simulink library "mylib"  (R2020a)
settings: Solver=VariableStepAuto  StartTime=0.0  StopTime=10.0  RelTol=1e-3
undefined symbols (not defined in the file): d_du_max_pu, dir_to_bus1, dir_to_bus_0L, dir_to_bus_2, dir_to_line1, dir_to_line_0L, dir_to_line_2, du_max_pu, du_ph_max_pu, Fi_0, Fi_T_H, Fi_T_L, Fi_T_M, I0_calc_0L, I0_comp_H, I0_comp_L, I0_comp_M, I0_max_0L, I2_max_2, I_diff1, I_diff2, I_diff3, I_diff4, I_diff5, I_diff_to, I_hight_CT1_G, I_hight_CT2_G, I_low_CT1, I_low_CT2, I_max1, I_max2, I_max3, I_max4, I_max5, I_min_sec_CT1, I_min_sec_CT2, I_unb, Iph_max_0L, Iph_max_2, jmp_in_zone, jmp_in_zone_0L, jmp_in_zone_2, K_dop, max_min1, only_K1_0L, only_K1_2, only_K2_0L, only_K2_2, only_K3_0L, only_K3_2, P_ctl_0, PQ_Fi_ctl_0, Q_ctl_0, S_set_0, set, set1, T_fast, T_I_ctl, T_off, T_on ... (+15)
libraries: $bdroot x184, powerlib_meascontrol x97
(part 11 of 14)

== system mylib/264_DZ_trans_st_v1/Poly12_det19_ph/Zc/stp_12 ==
  Y_in : Inport
  alg_in : Inport  Port=2
  Re_cur : Inport  Port=3
  Im_cur : Inport  Port=4
  Re_next : Inport  Port=5
  Im_next : Inport  Port=6
  re : Inport  Port=7
  im : Inport  Port=8
  start_pt : Inport  Port=9
  Re_start : Inport  Port=10
  Im_start : Inport  Port=11
  Constant : Constant  Value=0
  Constant1 : Constant  Value=0
  D1 : Logic  AllPortsSameDT=off  OutDataTypeStr=boolean
  Divide : Product  Inputs=**
  Divide1 : Product  Inputs=*/
  Logical Operator1 : Logic  Inputs=3  AllPortsSameDT=off  OutDataTypeStr=boolean
  Logical Operator2 : Logic  AllPortsSameDT=off  OutDataTypeStr=boolean
  Logical Operator3 : Logic  AllPortsSameDT=off  OutDataTypeStr=boolean
  Logical Operator4 : Logic  Operator=OR  AllPortsSameDT=off  OutDataTypeStr=boolean
  Logical Operator5 : Logic  AllPortsSameDT=off  OutDataTypeStr=boolean
  Logical Operator6 : Logic  Operator=OR  AllPortsSameDT=off  OutDataTypeStr=boolean
  Logical Operator7 : Logic  Operator=NOT  AllPortsSameDT=off  OutDataTypeStr=boolean
  Logical Operator8 : Logic  Operator=NOT  AllPortsSameDT=off  OutDataTypeStr=boolean
  Relational Operator{,1..3} (4 alike) : RelationalOperator  Operator===  OutDataTypeStr=boolean  RndMeth=Simplest
  Relational Operator4 : RelationalOperator  Operator=<  OutDataTypeStr=boolean  RndMeth=Simplest
  Relational Operator5 : RelationalOperator  Operator=>  OutDataTypeStr=boolean  RndMeth=Simplest
  Relational Operator6 : RelationalOperator  Operator=<  OutDataTypeStr=boolean  RndMeth=Simplest
  Relational Operator7 : RelationalOperator  Operator=>  OutDataTypeStr=boolean  RndMeth=Simplest
  Relational Operator8 : RelationalOperator  Operator=>  OutDataTypeStr=boolean  RndMeth=Simplest
  Switch{1..6} (6 alike) : Switch  Criteria=u2 > Threshold
  X2-X1 : Sum  Inputs=+-
  Y-Y1 : Sum  Inputs=+-
  Y2-Y1 : Sum  Inputs=+-
  Y2-Y2 : Sum
  Y_out : Outport
  alg_out : Outport  Port=2
  cur_Re : Outport  Port=3
  cur_Im : Outport  Port=4
  wires:
  Constant/1 -> Relational Operator1/2, Relational Operator/2
  Relational Operator1/1 -> D1/1
  Relational Operator/1 -> D1/2
  D1/1 -> Logical Operator1/1, Switch1/2, Switch2/2
  Re_next/1 -> Switch2/3, Relational Operator1/1
  Im_next/1 -> Switch1/3, Relational Operator/1
  Constant1/1 -> Relational Operator3/2, Relational Operator2/2
  Relational Operator2/1 -> Logical Operator1/3
  Relational Operator3/1 -> Logical Operator1/2
  Relational Operator4/1 -> Logical Operator2/1
  Relational Operator5/1 -> Logical Operator2/2
  Relational Operator6/1 -> Logical Operator3/1
  Relational Operator7/1 -> Logical Operator3/2
  Logical Operator2/1 -> Logical Operator4/1
  Logical Operator3/1 -> Logical Operator4/2
  Logical Operator4/1 -> Logical Operator5/1
  Logical Operator1/1 -> Logical Operator7/1
  Logical Operator7/1 -> Logical Operator6/1
  start_pt/1 -> Logical Operator6/2
  X2-X1/1 -> Divide/2
  Divide/1 -> Divide1/1
  Y2-Y1/1 -> Divide1/2
  Y-Y1/1 -> Divide/1
  Divide1/1 -> Y2-Y2/1
  Re_cur/1 -> Relational Operator3/1, X2-X1/2, Switch5/3, Y2-Y2/2
  Im_start/1 -> Switch1/1
  Re_start/1 -> Switch2/1
  re/1 -> Relational Operator8/2
  Y2-Y2/1 -> Relational Operator8/1
  im/1 -> Relational Operator7/1, Relational Operator6/1, Relational Operator5/1, Relational Operator4/1, Y-Y1/1
  Im_cur/1 -> Y2-Y1/2, Y-Y1/2, Relational Operator2/1, Switch6/3, Relational Operator6/2, Relational Operator5/2
  Switch2/1 -> X2-X1/1, Switch5/1
  Switch1/1 -> Y2-Y1/1, Switch6/1, Relational Operator7/2, Relational Operator4/2
  Relational Operator8/1 -> Logical Operator5/2
  Logical Operator5/1 -> Switch3/2
  Logical Operator6/1 -> Switch6/2, Switch5/2, Switch4/2
  Y_in/1 -> Switch4/3
  Switch3/1 -> alg_out/1, Switch4/1
  alg_in/1 -> Logical Operator8/1, Switch3/3
  Logical Operator8/1 -> Switch3/1
  Switch4/1 -> Y_out/1
  Switch6/1 -> cur_Im/1
  Switch5/1 -> cur_Re/1

== system mylib/264_DZ_trans_st_v1/Poly12_det19_ph/Zc/stp_2 ==
  Y_in : Inport
  alg_in : Inport  Port=2
  Re_cur : Inport  Port=3
  Im_cur : Inport  Port=4
  Re_next : Inport  Port=5
  Im_next : Inport  Port=6
  re : Inport  Port=7
  im : Inport  Port=8
  start_pt : Inport  Port=9
  Re_start : Inport  Port=10
  Im_start : Inport  Port=11
  Constant : Constant  Value=0
  Constant1 : Constant  Value=0
  D1 : Logic  AllPortsSameDT=off  OutDataTypeStr=boolean
  Divide : Product  Inputs=**
  Divide1 : Product  Inputs=*/
  Logical Operator1 : Logic  Inputs=3  AllPortsSameDT=off  OutDataTypeStr=boolean
  Logical Operator2 : Logic  AllPortsSameDT=off  OutDataTypeStr=boolean
  Logical Operator3 : Logic  AllPortsSameDT=off  OutDataTypeStr=boolean
  Logical Operator4 : Logic  Operator=OR  AllPortsSameDT=off  OutDataTypeStr=boolean
  Logical Operator5 : Logic  AllPortsSameDT=off  OutDataTypeStr=boolean
  Logical Operator6 : Logic  Operator=OR  AllPortsSameDT=off  OutDataTypeStr=boolean
  Logical Operator7 : Logic  Operator=NOT  AllPortsSameDT=off  OutDataTypeStr=boolean
  Logical Operator8 : Logic  Operator=NOT  AllPortsSameDT=off  OutDataTypeStr=boolean
  Relational Operator{,1..3} (4 alike) : RelationalOperator  Operator===  OutDataTypeStr=boolean  RndMeth=Simplest
  Relational Operator4 : RelationalOperator  Operator=<  OutDataTypeStr=boolean  RndMeth=Simplest
  Relational Operator5 : RelationalOperator  Operator=>  OutDataTypeStr=boolean  RndMeth=Simplest
  Relational Operator6 : RelationalOperator  Operator=<  OutDataTypeStr=boolean  RndMeth=Simplest
  Relational Operator7 : RelationalOperator  Operator=>  OutDataTypeStr=boolean  RndMeth=Simplest
  Relational Operator8 : RelationalOperator  Operator=>  OutDataTypeStr=boolean  RndMeth=Simplest
  Switch{1..6} (6 alike) : Switch  Criteria=u2 > Threshold
  X2-X1 : Sum  Inputs=+-
  Y-Y1 : Sum  Inputs=+-
  Y2-Y1 : Sum  Inputs=+-
  Y2-Y2 : Sum
  Y_out : Outport
  alg_out : Outport  Port=2
  cur_Re : Outport  Port=3
  cur_Im : Outport  Port=4
  wires:
  Constant/1 -> Relational Operator1/2, Relational Operator/2
  Relational Operator1/1 -> D1/1
  Relational Operator/1 -> D1/2
  D1/1 -> Logical Operator1/1, Switch1/2, Switch2/2
  Re_next/1 -> Switch2/3, Relational Operator1/1
  Im_next/1 -> Switch1/3, Relational Operator/1
  Constant1/1 -> Relational Operator3/2, Relational Operator2/2
  Relational Operator2/1 -> Logical Operator1/3
  Relational Operator3/1 -> Logical Operator1/2
  Relational Operator4/1 -> Logical Operator2/1
  Relational Operator5/1 -> Logical Operator2/2
  Relational Operator6/1 -> Logical Operator3/1
  Relational Operator7/1 -> Logical Operator3/2
  Logical Operator2/1 -> Logical Operator4/1
  Logical Operator3/1 -> Logical Operator4/2
  Logical Operator4/1 -> Logical Operator5/1
  Logical Operator1/1 -> Logical Operator7/1
  Logical Operator7/1 -> Logical Operator6/1
  start_pt/1 -> Logical Operator6/2
  X2-X1/1 -> Divide/2
  Divide/1 -> Divide1/1
  Y2-Y1/1 -> Divide1/2
  Y-Y1/1 -> Divide/1
  Divide1/1 -> Y2-Y2/1
  Re_cur/1 -> Relational Operator3/1, X2-X1/2, Switch5/3, Y2-Y2/2
  Im_start/1 -> Switch1/1
  Re_start/1 -> Switch2/1
  re/1 -> Relational Operator8/2
  Y2-Y2/1 -> Relational Operator8/1
  im/1 -> Relational Operator7/1, Relational Operator6/1, Relational Operator5/1, Relational Operator4/1, Y-Y1/1
  Im_cur/1 -> Y2-Y1/2, Y-Y1/2, Relational Operator2/1, Switch6/3, Relational Operator6/2, Relational Operator5/2
  Switch2/1 -> X2-X1/1, Switch5/1
  Switch1/1 -> Y2-Y1/1, Switch6/1, Relational Operator7/2, Relational Operator4/2
  Relational Operator8/1 -> Logical Operator5/2
  Logical Operator5/1 -> Switch3/2
  Logical Operator6/1 -> Switch6/2, Switch5/2, Switch4/2
  Y_in/1 -> Switch4/3
  Switch3/1 -> alg_out/1, Switch4/1
  alg_in/1 -> Logical Operator8/1, Switch3/3
  Logical Operator8/1 -> Switch3/1
  Switch4/1 -> Y_out/1
  Switch6/1 -> cur_Im/1
  Switch5/1 -> cur_Re/1

== system mylib/264_DZ_trans_st_v1/Poly12_det19_ph/Zc/stp_3 ==
  Y_in : Inport
  alg_in : Inport  Port=2
  Re_cur : Inport  Port=3
  Im_cur : Inport  Port=4
  Re_next : Inport  Port=5
  Im_next : Inport  Port=6
  re : Inport  Port=7
  im : Inport  Port=8
  start_pt : Inport  Port=9
  Re_start : Inport  Port=10
  Im_start : Inport  Port=11
  Constant : Constant  Value=0
  Constant1 : Constant  Value=0
  D1 : Logic  AllPortsSameDT=off  OutDataTypeStr=boolean
  Divide : Product  Inputs=**
  Divide1 : Product  Inputs=*/
  Logical Operator1 : Logic  Inputs=3  AllPortsSameDT=off  OutDataTypeStr=boolean
  Logical Operator2 : Logic  AllPortsSameDT=off  OutDataTypeStr=boolean
  Logical Operator3 : Logic  AllPortsSameDT=off  OutDataTypeStr=boolean
  Logical Operator4 : Logic  Operator=OR  AllPortsSameDT=off  OutDataTypeStr=boolean
  Logical Operator5 : Logic  AllPortsSameDT=off  OutDataTypeStr=boolean
  Logical Operator6 : Logic  Operator=OR  AllPortsSameDT=off  OutDataTypeStr=boolean
  Logical Operator7 : Logic  Operator=NOT  AllPortsSameDT=off  OutDataTypeStr=boolean
  Logical Operator8 : Logic  Operator=NOT  AllPortsSameDT=off  OutDataTypeStr=boolean
  Relational Operator{,1..3} (4 alike) : RelationalOperator  Operator===  OutDataTypeStr=boolean  RndMeth=Simplest
  Relational Operator4 : RelationalOperator  Operator=<  OutDataTypeStr=boolean  RndMeth=Simplest
  Relational Operator5 : RelationalOperator  Operator=>  OutDataTypeStr=boolean  RndMeth=Simplest
  Relational Operator6 : RelationalOperator  Operator=<  OutDataTypeStr=boolean  RndMeth=Simplest
  Relational Operator7 : RelationalOperator  Operator=>  OutDataTypeStr=boolean  RndMeth=Simplest
  Relational Operator8 : RelationalOperator  Operator=>  OutDataTypeStr=boolean  RndMeth=Simplest
  Switch{1..6} (6 alike) : Switch  Criteria=u2 > Threshold
  X2-X1 : Sum  Inputs=+-
  Y-Y1 : Sum  Inputs=+-
  Y2-Y1 : Sum  Inputs=+-
  Y2-Y2 : Sum
  Y_out : Outport
  alg_out : Outport  Port=2
  cur_Re : Outport  Port=3
  cur_Im : Outport  Port=4
  wires:
  Constant/1 -> Relational Operator1/2, Relational Operator/2
  Relational Operator1/1 -> D1/1
  Relational Operator/1 -> D1/2
  D1/1 -> Logical Operator1/1, Switch1/2, Switch2/2
  Re_next/1 -> Switch2/3, Relational Operator1/1
  Im_next/1 -> Switch1/3, Relational Operator/1
  Constant1/1 -> Relational Operator3/2, Relational Operator2/2
  Relational Operator2/1 -> Logical Operator1/3
  Relational Operator3/1 -> Logical Operator1/2
  Relational Operator4/1 -> Logical Operator2/1
  Relational Operator5/1 -> Logical Operator2/2
  Relational Operator6/1 -> Logical Operator3/1
  Relational Operator7/1 -> Logical Operator3/2
  Logical Operator2/1 -> Logical Operator4/1
  Logical Operator3/1 -> Logical Operator4/2
  Logical Operator4/1 -> Logical Operator5/1
  Logical Operator1/1 -> Logical Operator7/1
  Logical Operator7/1 -> Logical Operator6/1
  start_pt/1 -> Logical Operator6/2
  X2-X1/1 -> Divide/2
  Divide/1 -> Divide1/1
  Y2-Y1/1 -> Divide1/2
  Y-Y1/1 -> Divide/1
  Divide1/1 -> Y2-Y2/1
  Re_cur/1 -> Relational Operator3/1, X2-X1/2, Switch5/3, Y2-Y2/2
  Im_start/1 -> Switch1/1
  Re_start/1 -> Switch2/1
  re/1 -> Relational Operator8/2
  Y2-Y2/1 -> Relational Operator8/1
  im/1 -> Relational Operator7/1, Relational Operator6/1, Relational Operator5/1, Relational Operator4/1, Y-Y1/1
  Im_cur/1 -> Y2-Y1/2, Y-Y1/2, Relational Operator2/1, Switch6/3, Relational Operator6/2, Relational Operator5/2
  Switch2/1 -> X2-X1/1, Switch5/1
  Switch1/1 -> Y2-Y1/1, Switch6/1, Relational Operator7/2, Relational Operator4/2
  Relational Operator8/1 -> Logical Operator5/2
  Logical Operator5/1 -> Switch3/2
  Logical Operator6/1 -> Switch6/2, Switch5/2, Switch4/2
  Y_in/1 -> Switch4/3
  Switch3/1 -> alg_out/1, Switch4/1
  alg_in/1 -> Logical Operator8/1, Switch3/3
  Logical Operator8/1 -> Switch3/1
  Switch4/1 -> Y_out/1
  Switch6/1 -> cur_Im/1
  Switch5/1 -> cur_Re/1

== system mylib/264_DZ_trans_st_v1/Poly12_det19_ph/Zc/stp_4 ==
  Y_in : Inport
  alg_in : Inport  Port=2
  Re_cur : Inport  Port=3
  Im_cur : Inport  Port=4
  Re_next : Inport  Port=5
  Im_next : Inport  Port=6
  re : Inport  Port=7
  im : Inport  Port=8
  start_pt : Inport  Port=9
  Re_start : Inport  Port=10
  Im_start : Inport  Port=11
  Constant : Constant  Value=0
  Constant1 : Constant  Value=0
  D1 : Logic  AllPortsSameDT=off  OutDataTypeStr=boolean
  Divide : Product  Inputs=**
  Divide1 : Product  Inputs=*/
  Logical Operator1 : Logic  Inputs=3  AllPortsSameDT=off  OutDataTypeStr=boolean
  Logical Operator2 : Logic  AllPortsSameDT=off  OutDataTypeStr=boolean
  Logical Operator3 : Logic  AllPortsSameDT=off  OutDataTypeStr=boolean
  Logical Operator4 : Logic  Operator=OR  AllPortsSameDT=off  OutDataTypeStr=boolean
  Logical Operator5 : Logic  AllPortsSameDT=off  OutDataTypeStr=boolean
  Logical Operator6 : Logic  Operator=OR  AllPortsSameDT=off  OutDataTypeStr=boolean
  Logical Operator7 : Logic  Operator=NOT  AllPortsSameDT=off  OutDataTypeStr=boolean
  Logical Operator8 : Logic  Operator=NOT  AllPortsSameDT=off  OutDataTypeStr=boolean
  Relational Operator{,1..3} (4 alike) : RelationalOperator  Operator===  OutDataTypeStr=boolean  RndMeth=Simplest
  Relational Operator4 : RelationalOperator  Operator=<  OutDataTypeStr=boolean  RndMeth=Simplest
  Relational Operator5 : RelationalOperator  Operator=>  OutDataTypeStr=boolean  RndMeth=Simplest
  Relational Operator6 : RelationalOperator  Operator=<  OutDataTypeStr=boolean  RndMeth=Simplest
  Relational Operator7 : RelationalOperator  Operator=>  OutDataTypeStr=boolean  RndMeth=Simplest
  Relational Operator8 : RelationalOperator  Operator=>  OutDataTypeStr=boolean  RndMeth=Simplest
  Switch{1..6} (6 alike) : Switch  Criteria=u2 > Threshold
  X2-X1 : Sum  Inputs=+-
  Y-Y1 : Sum  Inputs=+-
  Y2-Y1 : Sum  Inputs=+-
  Y2-Y2 : Sum
  Y_out : Outport
  alg_out : Outport  Port=2
  cur_Re : Outport  Port=3
  cur_Im : Outport  Port=4
  wires:
  Constant/1 -> Relational Operator1/2, Relational Operator/2
  Relational Operator1/1 -> D1/1
  Relational Operator/1 -> D1/2
  D1/1 -> Logical Operator1/1, Switch1/2, Switch2/2
  Re_next/1 -> Switch2/3, Relational Operator1/1
  Im_next/1 -> Switch1/3, Relational Operator/1
  Constant1/1 -> Relational Operator3/2, Relational Operator2/2
  Relational Operator2/1 -> Logical Operator1/3
  Relational Operator3/1 -> Logical Operator1/2
  Relational Operator4/1 -> Logical Operator2/1
  Relational Operator5/1 -> Logical Operator2/2
  Relational Operator6/1 -> Logical Operator3/1
  Relational Operator7/1 -> Logical Operator3/2
  Logical Operator2/1 -> Logical Operator4/1
  Logical Operator3/1 -> Logical Operator4/2
  Logical Operator4/1 -> Logical Operator5/1
  Logical Operator1/1 -> Logical Operator7/1
  Logical Operator7/1 -> Logical Operator6/1
  start_pt/1 -> Logical Operator6/2
  X2-X1/1 -> Divide/2
  Divide/1 -> Divide1/1
  Y2-Y1/1 -> Divide1/2
  Y-Y1/1 -> Divide/1
  Divide1/1 -> Y2-Y2/1
  Re_cur/1 -> Relational Operator3/1, X2-X1/2, Switch5/3, Y2-Y2/2
  Im_start/1 -> Switch1/1
  Re_start/1 -> Switch2/1
  re/1 -> Relational Operator8/2
  Y2-Y2/1 -> Relational Operator8/1
  im/1 -> Relational Operator7/1, Relational Operator6/1, Relational Operator5/1, Relational Operator4/1, Y-Y1/1
  Im_cur/1 -> Y2-Y1/2, Y-Y1/2, Relational Operator2/1, Switch6/3, Relational Operator6/2, Relational Operator5/2
  Switch2/1 -> X2-X1/1, Switch5/1
  Switch1/1 -> Y2-Y1/1, Switch6/1, Relational Operator7/2, Relational Operator4/2
  Relational Operator8/1 -> Logical Operator5/2
  Logical Operator5/1 -> Switch3/2
  Logical Operator6/1 -> Switch6/2, Switch5/2, Switch4/2
  Y_in/1 -> Switch4/3
  Switch3/1 -> alg_out/1, Switch4/1
  alg_in/1 -> Logical Operator8/1, Switch3/3
  Logical Operator8/1 -> Switch3/1
  Switch4/1 -> Y_out/1
  Switch6/1 -> cur_Im/1
  Switch5/1 -> cur_Re/1

== system mylib/264_DZ_trans_st_v1/Poly12_det19_ph/Zc/stp_5 ==
  Y_in : Inport
  alg_in : Inport  Port=2
  Re_cur : Inport  Port=3
  Im_cur : Inport  Port=4
  Re_next : Inport  Port=5
  Im_next : Inport  Port=6
  re : Inport  Port=7
  im : Inport  Port=8
  start_pt : Inport  Port=9
  Re_start : Inport  Port=10
  Im_start : Inport  Port=11
  Constant : Constant  Value=0
  Constant1 : Constant  Value=0
  D1 : Logic  AllPortsSameDT=off  OutDataTypeStr=boolean
  Divide : Product  Inputs=**
  Divide1 : Product  Inputs=*/
  Logical Operator1 : Logic  Inputs=3  AllPortsSameDT=off  OutDataTypeStr=boolean
  Logical Operator2 : Logic  AllPortsSameDT=off  OutDataTypeStr=boolean
  Logical Operator3 : Logic  AllPortsSameDT=off  OutDataTypeStr=boolean
  Logical Operator4 : Logic  Operator=OR  AllPortsSameDT=off  OutDataTypeStr=boolean
  Logical Operator5 : Logic  AllPortsSameDT=off  OutDataTypeStr=boolean
  Logical Operator6 : Logic  Operator=OR  AllPortsSameDT=off  OutDataTypeStr=boolean
  Logical Operator7 : Logic  Operator=NOT  AllPortsSameDT=off  OutDataTypeStr=boolean
  Logical Operator8 : Logic  Operator=NOT  AllPortsSameDT=off  OutDataTypeStr=boolean
  Relational Operator{,1..3} (4 alike) : RelationalOperator  Operator===  OutDataTypeStr=boolean  RndMeth=Simplest
  Relational Operator4 : RelationalOperator  Operator=<  OutDataTypeStr=boolean  RndMeth=Simplest
  Relational Operator5 : RelationalOperator  Operator=>  OutDataTypeStr=boolean  RndMeth=Simplest
  Relational Operator6 : RelationalOperator  Operator=<  OutDataTypeStr=boolean  RndMeth=Simplest
  Relational Operator7 : RelationalOperator  Operator=>  OutDataTypeStr=boolean  RndMeth=Simplest
  Relational Operator8 : RelationalOperator  Operator=>  OutDataTypeStr=boolean  RndMeth=Simplest
  Switch{1..6} (6 alike) : Switch  Criteria=u2 > Threshold
  X2-X1 : Sum  Inputs=+-
  Y-Y1 : Sum  Inputs=+-
  Y2-Y1 : Sum  Inputs=+-
  Y2-Y2 : Sum
  Y_out : Outport
  alg_out : Outport  Port=2
  cur_Re : Outport  Port=3
  cur_Im : Outport  Port=4
  wires:
  Constant/1 -> Relational Operator1/2, Relational Operator/2
  Relational Operator1/1 -> D1/1
  Relational Operator/1 -> D1/2
  D1/1 -> Logical Operator1/1, Switch1/2, Switch2/2
  Re_next/1 -> Switch2/3, Relational Operator1/1
  Im_next/1 -> Switch1/3, Relational Operator/1
  Constant1/1 -> Relational Operator3/2, Relational Operator2/2
  Relational Operator2/1 -> Logical Operator1/3
  Relational Operator3/1 -> Logical Operator1/2
  Relational Operator4/1 -> Logical Operator2/1
  Relational Operator5/1 -> Logical Operator2/2
  Relational Operator6/1 -> Logical Operator3/1
  Relational Operator7/1 -> Logical Operator3/2
  Logical Operator2/1 -> Logical Operator4/1
  Logical Operator3/1 -> Logical Operator4/2
  Logical Operator4/1 -> Logical Operator5/1
  Logical Operator1/1 -> Logical Operator7/1
  Logical Operator7/1 -> Logical Operator6/1
  start_pt/1 -> Logical Operator6/2
  X2-X1/1 -> Divide/2
  Divide/1 -> Divide1/1
  Y2-Y1/1 -> Divide1/2
  Y-Y1/1 -> Divide/1
  Divide1/1 -> Y2-Y2/1
  Re_cur/1 -> Relational Operator3/1, X2-X1/2, Switch5/3, Y2-Y2/2
  Im_start/1 -> Switch1/1
  Re_start/1 -> Switch2/1
  re/1 -> Relational Operator8/2
  Y2-Y2/1 -> Relational Operator8/1
  im/1 -> Relational Operator7/1, Relational Operator6/1, Relational Operator5/1, Relational Operator4/1, Y-Y1/1
  Im_cur/1 -> Y2-Y1/2, Y-Y1/2, Relational Operator2/1, Switch6/3, Relational Operator6/2, Relational Operator5/2
  Switch2/1 -> X2-X1/1, Switch5/1
  Switch1/1 -> Y2-Y1/1, Switch6/1, Relational Operator7/2, Relational Operator4/2
  Relational Operator8/1 -> Logical Operator5/2
  Logical Operator5/1 -> Switch3/2
  Logical Operator6/1 -> Switch6/2, Switch5/2, Switch4/2
  Y_in/1 -> Switch4/3
  Switch3/1 -> alg_out/1, Switch4/1
  alg_in/1 -> Logical Operator8/1, Switch3/3
  Logical Operator8/1 -> Switch3/1
  Switch4/1 -> Y_out/1
  Switch6/1 -> cur_Im/1
  Switch5/1 -> cur_Re/1

== system mylib/264_DZ_trans_st_v1/Poly12_det19_ph/Zc/stp_6 ==
  Y_in : Inport
  alg_in : Inport  Port=2
  Re_cur : Inport  Port=3
  Im_cur : Inport  Port=4
  Re_next : Inport  Port=5
  Im_next : Inport  Port=6
  re : Inport  Port=7
  im : Inport  Port=8
  start_pt : Inport  Port=9
  Re_start : Inport  Port=10
  Im_start : Inport  Port=11
  Constant : Constant  Value=0
  Constant1 : Constant  Value=0
  D1 : Logic  AllPortsSameDT=off  OutDataTypeStr=boolean
  Divide : Product  Inputs=**
  Divide1 : Product  Inputs=*/
  Logical Operator1 : Logic  Inputs=3  AllPortsSameDT=off  OutDataTypeStr=boolean
  Logical Operator2 : Logic  AllPortsSameDT=off  OutDataTypeStr=boolean
  Logical Operator3 : Logic  AllPortsSameDT=off  OutDataTypeStr=boolean
  Logical Operator4 : Logic  Operator=OR  AllPortsSameDT=off  OutDataTypeStr=boolean
  Logical Operator5 : Logic  AllPortsSameDT=off  OutDataTypeStr=boolean
  Logical Operator6 : Logic  Operator=OR  AllPortsSameDT=off  OutDataTypeStr=boolean
  Logical Operator7 : Logic  Operator=NOT  AllPortsSameDT=off  OutDataTypeStr=boolean
  Logical Operator8 : Logic  Operator=NOT  AllPortsSameDT=off  OutDataTypeStr=boolean
  Relational Operator{,1..3} (4 alike) : RelationalOperator  Operator===  OutDataTypeStr=boolean  RndMeth=Simplest
  Relational Operator4 : RelationalOperator  Operator=<  OutDataTypeStr=boolean  RndMeth=Simplest
  Relational Operator5 : RelationalOperator  Operator=>  OutDataTypeStr=boolean  RndMeth=Simplest
  Relational Operator6 : RelationalOperator  Operator=<  OutDataTypeStr=boolean  RndMeth=Simplest
  Relational Operator7 : RelationalOperator  Operator=>  OutDataTypeStr=boolean  RndMeth=Simplest
  Relational Operator8 : RelationalOperator  Operator=>  OutDataTypeStr=boolean  RndMeth=Simplest
  Switch{1..6} (6 alike) : Switch  Criteria=u2 > Threshold
  X2-X1 : Sum  Inputs=+-
  Y-Y1 : Sum  Inputs=+-
  Y2-Y1 : Sum  Inputs=+-
  Y2-Y2 : Sum
  Y_out : Outport
  alg_out : Outport  Port=2
  cur_Re : Outport  Port=3
  cur_Im : Outport  Port=4
  wires:
  Constant/1 -> Relational Operator1/2, Relational Operator/2
  Relational Operator1/1 -> D1/1
  Relational Operator/1 -> D1/2
  D1/1 -> Logical Operator1/1, Switch1/2, Switch2/2
  Re_next/1 -> Switch2/3, Relational Operator1/1
  Im_next/1 -> Switch1/3, Relational Operator/1
  Constant1/1 -> Relational Operator3/2, Relational Operator2/2
  Relational Operator2/1 -> Logical Operator1/3
  Relational Operator3/1 -> Logical Operator1/2
  Relational Operator4/1 -> Logical Operator2/1
  Relational Operator5/1 -> Logical Operator2/2
  Relational Operator6/1 -> Logical Operator3/1
  Relational Operator7/1 -> Logical Operator3/2
  Logical Operator2/1 -> Logical Operator4/1
  Logical Operator3/1 -> Logical Operator4/2
  Logical Operator4/1 -> Logical Operator5/1
  Logical Operator1/1 -> Logical Operator7/1
  Logical Operator7/1 -> Logical Operator6/1
  start_pt/1 -> Logical Operator6/2
  X2-X1/1 -> Divide/2
  Divide/1 -> Divide1/1
  Y2-Y1/1 -> Divide1/2
  Y-Y1/1 -> Divide/1
  Divide1/1 -> Y2-Y2/1
  Re_cur/1 -> Relational Operator3/1, X2-X1/2, Switch5/3, Y2-Y2/2
  Im_start/1 -> Switch1/1
  Re_start/1 -> Switch2/1
  re/1 -> Relational Operator8/2
  Y2-Y2/1 -> Relational Operator8/1
  im/1 -> Relational Operator7/1, Relational Operator6/1, Relational Operator5/1, Relational Operator4/1, Y-Y1/1
  Im_cur/1 -> Y2-Y1/2, Y-Y1/2, Relational Operator2/1, Switch6/3, Relational Operator6/2, Relational Operator5/2
  Switch2/1 -> X2-X1/1, Switch5/1
  Switch1/1 -> Y2-Y1/1, Switch6/1, Relational Operator7/2, Relational Operator4/2
  Relational Operator8/1 -> Logical Operator5/2
  Logical Operator5/1 -> Switch3/2
  Logical Operator6/1 -> Switch6/2, Switch5/2, Switch4/2
  Y_in/1 -> Switch4/3
  Switch3/1 -> alg_out/1, Switch4/1
  alg_in/1 -> Logical Operator8/1, Switch3/3
  Logical Operator8/1 -> Switch3/1
  Switch4/1 -> Y_out/1
  Switch6/1 -> cur_Im/1
  Switch5/1 -> cur_Re/1

== system mylib/264_DZ_trans_st_v1/Poly12_det19_ph/Zc/stp_7 ==
  Y_in : Inport
  alg_in : Inport  Port=2
  Re_cur : Inport  Port=3
  Im_cur : Inport  Port=4
  Re_next : Inport  Port=5
  Im_next : Inport  Port=6
  re : Inport  Port=7
  im : Inport  Port=8
  start_pt : Inport  Port=9
  Re_start : Inport  Port=10
  Im_start : Inport  Port=11
  Constant : Constant  Value=0
  Constant1 : Constant  Value=0
  D1 : Logic  AllPortsSameDT=off  OutDataTypeStr=boolean
  Divide : Product  Inputs=**
  Divide1 : Product  Inputs=*/
  Logical Operator1 : Logic  Inputs=3  AllPortsSameDT=off  OutDataTypeStr=boolean
  Logical Operator2 : Logic  AllPortsSameDT=off  OutDataTypeStr=boolean
  Logical Operator3 : Logic  AllPortsSameDT=off  OutDataTypeStr=boolean
  Logical Operator4 : Logic  Operator=OR  AllPortsSameDT=off  OutDataTypeStr=boolean
  Logical Operator5 : Logic  AllPortsSameDT=off  OutDataTypeStr=boolean
  Logical Operator6 : Logic  Operator=OR  AllPortsSameDT=off  OutDataTypeStr=boolean
  Logical Operator7 : Logic  Operator=NOT  AllPortsSameDT=off  OutDataTypeStr=boolean
  Logical Operator8 : Logic  Operator=NOT  AllPortsSameDT=off  OutDataTypeStr=boolean
  Relational Operator{,1..3} (4 alike) : RelationalOperator  Operator===  OutDataTypeStr=boolean  RndMeth=Simplest
  Relational Operator4 : RelationalOperator  Operator=<  OutDataTypeStr=boolean  RndMeth=Simplest
  Relational Operator5 : RelationalOperator  Operator=>  OutDataTypeStr=boolean  RndMeth=Simplest
  Relational Operator6 : RelationalOperator  Operator=<  OutDataTypeStr=boolean  RndMeth=Simplest
  Relational Operator7 : RelationalOperator  Operator=>  OutDataTypeStr=boolean  RndMeth=Simplest
  Relational Operator8 : RelationalOperator  Operator=>  OutDataTypeStr=boolean  RndMeth=Simplest
  Switch{1..6} (6 alike) : Switch  Criteria=u2 > Threshold
  X2-X1 : Sum  Inputs=+-
  Y-Y1 : Sum  Inputs=+-
  Y2-Y1 : Sum  Inputs=+-
  Y2-Y2 : Sum
  Y_out : Outport
  alg_out : Outport  Port=2
  cur_Re : Outport  Port=3
  cur_Im : Outport  Port=4
  wires:
  Constant/1 -> Relational Operator1/2, Relational Operator/2
  Relational Operator1/1 -> D1/1
  Relational Operator/1 -> D1/2
  D1/1 -> Logical Operator1/1, Switch1/2, Switch2/2
  Re_next/1 -> Switch2/3, Relational Operator1/1
  Im_next/1 -> Switch1/3, Relational Operator/1
  Constant1/1 -> Relational Operator3/2, Relational Operator2/2
  Relational Operator2/1 -> Logical Operator1/3
  Relational Operator3/1 -> Logical Operator1/2
  Relational Operator4/1 -> Logical Operator2/1
  Relational Operator5/1 -> Logical Operator2/2
  Relational Operator6/1 -> Logical Operator3/1
  Relational Operator7/1 -> Logical Operator3/2
  Logical Operator2/1 -> Logical Operator4/1
  Logical Operator3/1 -> Logical Operator4/2
  Logical Operator4/1 -> Logical Operator5/1
  Logical Operator1/1 -> Logical Operator7/1
  Logical Operator7/1 -> Logical Operator6/1
  start_pt/1 -> Logical Operator6/2
  X2-X1/1 -> Divide/2
  Divide/1 -> Divide1/1
  Y2-Y1/1 -> Divide1/2
  Y-Y1/1 -> Divide/1
  Divide1/1 -> Y2-Y2/1
  Re_cur/1 -> Relational Operator3/1, X2-X1/2, Switch5/3, Y2-Y2/2
  Im_start/1 -> Switch1/1
  Re_start/1 -> Switch2/1
  re/1 -> Relational Operator8/2
  Y2-Y2/1 -> Relational Operator8/1
  im/1 -> Relational Operator7/1, Relational Operator6/1, Relational Operator5/1, Relational Operator4/1, Y-Y1/1
  Im_cur/1 -> Y2-Y1/2, Y-Y1/2, Relational Operator2/1, Switch6/3, Relational Operator6/2, Relational Operator5/2
  Switch2/1 -> X2-X1/1, Switch5/1
  Switch1/1 -> Y2-Y1/1, Switch6/1, Relational Operator7/2, Relational Operator4/2
  Relational Operator8/1 -> Logical Operator5/2
  Logical Operator5/1 -> Switch3/2
  Logical Operator6/1 -> Switch6/2, Switch5/2, Switch4/2
  Y_in/1 -> Switch4/3
  Switch3/1 -> alg_out/1, Switch4/1
  alg_in/1 -> Logical Operator8/1, Switch3/3
  Logical Operator8/1 -> Switch3/1
  Switch4/1 -> Y_out/1
  Switch6/1 -> cur_Im/1
  Switch5/1 -> cur_Re/1

== system mylib/264_DZ_trans_st_v1/Poly12_det19_ph/Zc/stp_8 ==
  Y_in : Inport
  alg_in : Inport  Port=2
  Re_cur : Inport  Port=3
  Im_cur : Inport  Port=4
  Re_next : Inport  Port=5
  Im_next : Inport  Port=6
  re : Inport  Port=7
  im : Inport  Port=8
  start_pt : Inport  Port=9
  Re_start : Inport  Port=10
  Im_start : Inport  Port=11
  Constant : Constant  Value=0
  Constant1 : Constant  Value=0
  D1 : Logic  AllPortsSameDT=off  OutDataTypeStr=boolean
  Divide : Product  Inputs=**
  Divide1 : Product  Inputs=*/
  Logical Operator1 : Logic  Inputs=3  AllPortsSameDT=off  OutDataTypeStr=boolean
  Logical Operator2 : Logic  AllPortsSameDT=off  OutDataTypeStr=boolean
  Logical Operator3 : Logic  AllPortsSameDT=off  OutDataTypeStr=boolean
  Logical Operator4 : Logic  Operator=OR  AllPortsSameDT=off  OutDataTypeStr=boolean
  Logical Operator5 : Logic  AllPortsSameDT=off  OutDataTypeStr=boolean
  Logical Operator6 : Logic  Operator=OR  AllPortsSameDT=off  OutDataTypeStr=boolean
  Logical Operator7 : Logic  Operator=NOT  AllPortsSameDT=off  OutDataTypeStr=boolean
  Logical Operator8 : Logic  Operator=NOT  AllPortsSameDT=off  OutDataTypeStr=boolean
  Relational Operator{,1..3} (4 alike) : RelationalOperator  Operator===  OutDataTypeStr=boolean  RndMeth=Simplest
  Relational Operator4 : RelationalOperator  Operator=<  OutDataTypeStr=boolean  RndMeth=Simplest
  Relational Operator5 : RelationalOperator  Operator=>  OutDataTypeStr=boolean  RndMeth=Simplest
  Relational Operator6 : RelationalOperator  Operator=<  OutDataTypeStr=boolean  RndMeth=Simplest
  Relational Operator7 : RelationalOperator  Operator=>  OutDataTypeStr=boolean  RndMeth=Simplest
  Relational Operator8 : RelationalOperator  Operator=>  OutDataTypeStr=boolean  RndMeth=Simplest
  Switch{1..6} (6 alike) : Switch  Criteria=u2 > Threshold
  X2-X1 : Sum  Inputs=+-
  Y-Y1 : Sum  Inputs=+-
  Y2-Y1 : Sum  Inputs=+-
  Y2-Y2 : Sum
  Y_out : Outport
  alg_out : Outport  Port=2
  cur_Re : Outport  Port=3
  cur_Im : Outport  Port=4
  wires:
  Constant/1 -> Relational Operator1/2, Relational Operator/2
  Relational Operator1/1 -> D1/1
  Relational Operator/1 -> D1/2
  D1/1 -> Logical Operator1/1, Switch1/2, Switch2/2
  Re_next/1 -> Switch2/3, Relational Operator1/1
  Im_next/1 -> Switch1/3, Relational Operator/1
  Constant1/1 -> Relational Operator3/2, Relational Operator2/2
  Relational Operator2/1 -> Logical Operator1/3
  Relational Operator3/1 -> Logical Operator1/2
  Relational Operator4/1 -> Logical Operator2/1
  Relational Operator5/1 -> Logical Operator2/2
  Relational Operator6/1 -> Logical Operator3/1
  Relational Operator7/1 -> Logical Operator3/2
  Logical Operator2/1 -> Logical Operator4/1
  Logical Operator3/1 -> Logical Operator4/2
  Logical Operator4/1 -> Logical Operator5/1
  Logical Operator1/1 -> Logical Operator7/1
  Logical Operator7/1 -> Logical Operator6/1
  start_pt/1 -> Logical Operator6/2
  X2-X1/1 -> Divide/2
  Divide/1 -> Divide1/1
  Y2-Y1/1 -> Divide1/2
  Y-Y1/1 -> Divide/1
  Divide1/1 -> Y2-Y2/1
  Re_cur/1 -> Relational Operator3/1, X2-X1/2, Switch5/3, Y2-Y2/2
  Im_start/1 -> Switch1/1
  Re_start/1 -> Switch2/1
  re/1 -> Relational Operator8/2
  Y2-Y2/1 -> Relational Operator8/1
  im/1 -> Relational Operator7/1, Relational Operator6/1, Relational Operator5/1, Relational Operator4/1, Y-Y1/1
  Im_cur/1 -> Y2-Y1/2, Y-Y1/2, Relational Operator2/1, Switch6/3, Relational Operator6/2, Relational Operator5/2
  Switch2/1 -> X2-X1/1, Switch5/1
  Switch1/1 -> Y2-Y1/1, Switch6/1, Relational Operator7/2, Relational Operator4/2
  Relational Operator8/1 -> Logical Operator5/2
  Logical Operator5/1 -> Switch3/2
  Logical Operator6/1 -> Switch6/2, Switch5/2, Switch4/2
  Y_in/1 -> Switch4/3
  Switch3/1 -> alg_out/1, Switch4/1
  alg_in/1 -> Logical Operator8/1, Switch3/3
  Logical Operator8/1 -> Switch3/1
  Switch4/1 -> Y_out/1
  Switch6/1 -> cur_Im/1
  Switch5/1 -> cur_Re/1

== system mylib/264_DZ_trans_st_v1/Poly12_det19_ph/Zc/stp_9 ==
  Y_in : Inport
  alg_in : Inport  Port=2
  Re_cur : Inport  Port=3
  Im_cur : Inport  Port=4
  Re_next : Inport  Port=5
  Im_next : Inport  Port=6
  re : Inport  Port=7
  im : Inport  Port=8
  start_pt : Inport  Port=9
  Re_start : Inport  Port=10
  Im_start : Inport  Port=11
  Constant : Constant  Value=0
  Constant1 : Constant  Value=0
  D1 : Logic  AllPortsSameDT=off  OutDataTypeStr=boolean
  Divide : Product  Inputs=**
  Divide1 : Product  Inputs=*/
  Logical Operator1 : Logic  Inputs=3  AllPortsSameDT=off  OutDataTypeStr=boolean
  Logical Operator2 : Logic  AllPortsSameDT=off  OutDataTypeStr=boolean
  Logical Operator3 : Logic  AllPortsSameDT=off  OutDataTypeStr=boolean
  Logical Operator4 : Logic  Operator=OR  AllPortsSameDT=off  OutDataTypeStr=boolean
  Logical Operator5 : Logic  AllPortsSameDT=off  OutDataTypeStr=boolean
  Logical Operator6 : Logic  Operator=OR  AllPortsSameDT=off  OutDataTypeStr=boolean
  Logical Operator7 : Logic  Operator=NOT  AllPortsSameDT=off  OutDataTypeStr=boolean
  Logical Operator8 : Logic  Operator=NOT  AllPortsSameDT=off  OutDataTypeStr=boolean
  Relational Operator{,1..3} (4 alike) : RelationalOperator  Operator===  OutDataTypeStr=boolean  RndMeth=Simplest
  Relational Operator4 : RelationalOperator  Operator=<  OutDataTypeStr=boolean  RndMeth=Simplest
  Relational Operator5 : RelationalOperator  Operator=>  OutDataTypeStr=boolean  RndMeth=Simplest
  Relational Operator6 : RelationalOperator  Operator=<  OutDataTypeStr=boolean  RndMeth=Simplest
  Relational Operator7 : RelationalOperator  Operator=>  OutDataTypeStr=boolean  RndMeth=Simplest
  Relational Operator8 : RelationalOperator  Operator=>  OutDataTypeStr=boolean  RndMeth=Simplest
  Switch{1..6} (6 alike) : Switch  Criteria=u2 > Threshold
  X2-X1 : Sum  Inputs=+-
  Y-Y1 : Sum  Inputs=+-
  Y2-Y1 : Sum  Inputs=+-
  Y2-Y2 : Sum
  Y_out : Outport
  alg_out : Outport  Port=2
  cur_Re : Outport  Port=3
  cur_Im : Outport  Port=4
  wires:
  Constant/1 -> Relational Operator1/2, Relational Operator/2
  Relational Operator1/1 -> D1/1
  Relational Operator/1 -> D1/2
  D1/1 -> Logical Operator1/1, Switch1/2, Switch2/2
  Re_next/1 -> Switch2/3, Relational Operator1/1
  Im_next/1 -> Switch1/3, Relational Operator/1
  Constant1/1 -> Relational Operator3/2, Relational Operator2/2
  Relational Operator2/1 -> Logical Operator1/3
  Relational Operator3/1 -> Logical Operator1/2
  Relational Operator4/1 -> Logical Operator2/1
  Relational Operator5/1 -> Logical Operator2/2
  Relational Operator6/1 -> Logical Operator3/1
  Relational Operator7/1 -> Logical Operator3/2
  Logical Operator2/1 -> Logical Operator4/1
  Logical Operator3/1 -> Logical Operator4/2
  Logical Operator4/1 -> Logical Operator5/1
  Logical Operator1/1 -> Logical Operator7/1
  Logical Operator7/1 -> Logical Operator6/1
  start_pt/1 -> Logical Operator6/2
  X2-X1/1 -> Divide/2
  Divide/1 -> Divide1/1
  Y2-Y1/1 -> Divide1/2
  Y-Y1/1 -> Divide/1
  Divide1/1 -> Y2-Y2/1
  Re_cur/1 -> Relational Operator3/1, X2-X1/2, Switch5/3, Y2-Y2/2
  Im_start/1 -> Switch1/1
  Re_start/1 -> Switch2/1
  re/1 -> Relational Operator8/2
  Y2-Y2/1 -> Relational Operator8/1
  im/1 -> Relational Operator7/1, Relational Operator6/1, Relational Operator5/1, Relational Operator4/1, Y-Y1/1
  Im_cur/1 -> Y2-Y1/2, Y-Y1/2, Relational Operator2/1, Switch6/3, Relational Operator6/2, Relational Operator5/2
  Switch2/1 -> X2-X1/1, Switch5/1
  Switch1/1 -> Y2-Y1/1, Switch6/1, Relational Operator7/2, Relational Operator4/2
  Relational Operator8/1 -> Logical Operator5/2
  Logical Operator5/1 -> Switch3/2
  Logical Operator6/1 -> Switch6/2, Switch5/2, Switch4/2
  Y_in/1 -> Switch4/3
  Switch3/1 -> alg_out/1, Switch4/1
  alg_in/1 -> Logical Operator8/1, Switch3/3
  Logical Operator8/1 -> Switch3/1
  Switch4/1 -> Y_out/1
  Switch6/1 -> cur_Im/1
  Switch5/1 -> cur_Re/1

== system mylib/264_DZ_trans_st_v1/z_calc_ph_line19/Z_comp/Z_a ==
  U_re : Inport
  U_im : Inport  Port=2
  I_re : Inport  Port=3
  I_im : Inport  Port=4
  I0_re : Inport  Port=5
  I0_im : Inport  Port=6
  I0_re_prl : Inport  Port=7
  I0_im_prl : Inport  Port=8
  K_I0_re : Inport  Port=9
  K_I0_im : Inport  Port=10
  K_I0_prl_re : Inport  Port=11
  K_I0_prl_im : Inport  Port=12
  Add{,1..3} (4 alike) : Sum
  Constant : Constant  Value=3
  Constant1 : Constant  Value=3
  Divide{,1..3} (4 alike) : Product  Inputs=**
  Iph_add_3I0K : $bdroot/orto_MUL_orto  SystemSampleTime=-1  Latency=0  AutoFrameSizeCalculation=off
  Iph_add_3I0K1 : $bdroot/orto_MUL_orto  SystemSampleTime=-1  Latency=0  AutoFrameSizeCalculation=off
  ORTOTOMODULE : $bdroot/ORTOTOMODULE  SystemSampleTime=-1  Latency=0  AutoFrameSizeCalculation=off
  ORTOTOMODULE1 : $bdroot/ORTOTOMODULE  SystemSampleTime=-1  Latency=0  AutoFrameSizeCalculation=off
  orto_DIV_orto : $bdroot/orto_DIV_orto  SystemSampleTime=-1  Latency=0  AutoFrameSizeCalculation=off
  orto_DIV_orto1 : $bdroot/orto_DIV_orto  SystemSampleTime=-1  Latency=0  AutoFrameSizeCalculation=off
  R_comp : Outport
  R : Outport  Port=2
  X_comp : Outport  Port=3
  X : Outport  Port=4
  Z_comp : Outport  Port=5
  Z : Outport  Port=6
  wires:
  Constant/1 -> Divide3/2, Divide2/2
  Constant1/1 -> Divide/2, Divide1/2
  I0_re/1 -> Divide/1
  I0_im/1 -> Divide1/1
  I0_re_prl/1 -> Divide2/1
  I0_im_prl/1 -> Divide3/1
  K_I0_prl_re/1 -> Iph_add_3I0K1/3
  K_I0_prl_im/1 -> Iph_add_3I0K1/4
  K_I0_re/1 -> Iph_add_3I0K/3
  K_I0_im/1 -> Iph_add_3I0K/4
  Divide3/1 -> Iph_add_3I0K1/2
  Divide2/1 -> Iph_add_3I0K1/1
  Divide1/1 -> Iph_add_3I0K/2
  Divide/1 -> Iph_add_3I0K/1
  Iph_add_3I0K/1 -> Add/2
  Iph_add_3I0K/2 -> Add1/2
  Add/1 -> Add2/1
  Iph_add_3I0K1/1 -> Add2/2
  Iph_add_3I0K1/2 -> Add3/2
  Add1/1 -> Add3/1
  I_im/1 -> orto_DIV_orto/4, Add1/1
  I_re/1 -> orto_DIV_orto/3, Add/1
  U_re/1 -> orto_DIV_orto1/1, orto_DIV_orto/1
  U_im/1 -> orto_DIV_orto1/2, orto_DIV_orto/2
  Add3/1 -> orto_DIV_orto1/4
  Add2/1 -> orto_DIV_orto1/3
  orto_DIV_orto1/2 -> X_comp/1, ORTOTOMODULE/2
  orto_DIV_orto1/1 -> R_comp/1, ORTOTOMODULE/1
  orto_DIV_orto/2 -> X/1, ORTOTOMODULE1/2
  orto_DIV_orto/1 -> R/1, ORTOTOMODULE1/1
  ORTOTOMODULE/1 -> Z_comp/1
  ORTOTOMODULE1/1 -> Z/1

== system mylib/264_DZ_trans_st_v1/z_calc_ph_line19/Z_comp/Z_b ==
  U_re : Inport
  U_im : Inport  Port=2
  I_re : Inport  Port=3
  I_im : Inport  Port=4
  I0_re : Inport  Port=5
  I0_im : Inport  Port=6
  I0_re_prl : Inport  Port=7
  I0_im_prl : Inport  Port=8
  K_I0_re : Inport  Port=9
  K_I0_im : Inport  Port=10
  K_I0_prl_re : Inport  Port=11
  K_I0_prl_im : Inport  Port=12
  Add{,1..3} (4 alike) : Sum
  Constant : Constant  Value=3
  Constant1 : Constant  Value=3
  Divide{,1..3} (4 alike) : Product  Inputs=**
  Iph_add_3I0K : $bdroot/orto_MUL_orto  SystemSampleTime=-1  Latency=0  AutoFrameSizeCalculation=off
  Iph_add_3I0K1 : $bdroot/orto_MUL_orto  SystemSampleTime=-1  Latency=0  AutoFrameSizeCalculation=off
  ORTOTOMODULE : $bdroot/ORTOTOMODULE  SystemSampleTime=-1  Latency=0  AutoFrameSizeCalculation=off
  ORTOTOMODULE1 : $bdroot/ORTOTOMODULE  SystemSampleTime=-1  Latency=0  AutoFrameSizeCalculation=off
  orto_DIV_orto : $bdroot/orto_DIV_orto  SystemSampleTime=-1  Latency=0  AutoFrameSizeCalculation=off
  orto_DIV_orto1 : $bdroot/orto_DIV_orto  SystemSampleTime=-1  Latency=0  AutoFrameSizeCalculation=off
  R_comp : Outport
  R : Outport  Port=2
  X_comp : Outport  Port=3
  X : Outport  Port=4
  Z_comp : Outport  Port=5
  Z : Outport  Port=6
  wires:
  Constant/1 -> Divide3/2, Divide2/2
  Constant1/1 -> Divide/2, Divide1/2
  I0_re/1 -> Divide/1
  I0_im/1 -> Divide1/1
  I0_re_prl/1 -> Divide2/1
  I0_im_prl/1 -> Divide3/1
  K_I0_prl_re/1 -> Iph_add_3I0K1/3
  K_I0_prl_im/1 -> Iph_add_3I0K1/4
  K_I0_re/1 -> Iph_add_3I0K/3
  K_I0_im/1 -> Iph_add_3I0K/4
  Divide3/1 -> Iph_add_3I0K1/2
  Divide2/1 -> Iph_add_3I0K1/1
  Divide1/1 -> Iph_add_3I0K/2
  Divide/1 -> Iph_add_3I0K/1
  Iph_add_3I0K/1 -> Add/2
  Iph_add_3I0K/2 -> Add1/2
  Add/1 -> Add2/1
  Iph_add_3I0K1/1 -> Add2/2
  Iph_add_3I0K1/2 -> Add3/2
  Add1/1 -> Add3/1
  I_im/1 -> orto_DIV_orto/4, Add1/1
  I_re/1 -> orto_DIV_orto/3, Add/1
  U_re/1 -> orto_DIV_orto1/1, orto_DIV_orto/1
  U_im/1 -> orto_DIV_orto1/2, orto_DIV_orto/2
  Add3/1 -> orto_DIV_orto1/4
  Add2/1 -> orto_DIV_orto1/3
  orto_DIV_orto1/2 -> X_comp/1, ORTOTOMODULE/2
  orto_DIV_orto1/1 -> R_comp/1, ORTOTOMODULE/1
  orto_DIV_orto/2 -> X/1, ORTOTOMODULE1/2
  orto_DIV_orto/1 -> R/1, ORTOTOMODULE1/1
  ORTOTOMODULE/1 -> Z_comp/1
  ORTOTOMODULE1/1 -> Z/1

== system mylib/264_DZ_trans_st_v1/z_calc_ph_line19/Z_comp/Z_c ==
  U_re : Inport
  U_im : Inport  Port=2
  I_re : Inport  Port=3
  I_im : Inport  Port=4
  I0_re : Inport  Port=5
  I0_im : Inport  Port=6
  I0_re_prl : Inport  Port=7
  I0_im_prl : Inport  Port=8
  K_I0_re : Inport  Port=9
  K_I0_im : Inport  Port=10
  K_I0_prl_re : Inport  Port=11
  K_I0_prl_im : Inport  Port=12
  Add{,1..3} (4 alike) : Sum
  Constant : Constant  Value=3
  Constant1 : Constant  Value=3
  Divide{,1..3} (4 alike) : Product  Inputs=**
  Iph_add_3I0K : $bdroot/orto_MUL_orto  SystemSampleTime=-1  Latency=0  AutoFrameSizeCalculation=off
  Iph_add_3I0K1 : $bdroot/orto_MUL_orto  SystemSampleTime=-1  Latency=0  AutoFrameSizeCalculation=off
  ORTOTOMODULE : $bdroot/ORTOTOMODULE  SystemSampleTime=-1  Latency=0  AutoFrameSizeCalculation=off
  ORTOTOMODULE1 : $bdroot/ORTOTOMODULE  SystemSampleTime=-1  Latency=0  AutoFrameSizeCalculation=off
  orto_DIV_orto : $bdroot/orto_DIV_orto  SystemSampleTime=-1  Latency=0  AutoFrameSizeCalculation=off
  orto_DIV_orto1 : $bdroot/orto_DIV_orto  SystemSampleTime=-1  Latency=0  AutoFrameSizeCalculation=off
  R_comp : Outport
  R : Outport  Port=2
  X_comp : Outport  Port=3
  X : Outport  Port=4
  Z_comp : Outport  Port=5
  Z : Outport  Port=6
  wires:
  Constant/1 -> Divide3/2, Divide2/2
  Constant1/1 -> Divide/2, Divide1/2
  I0_re/1 -> Divide/1
  I0_im/1 -> Divide1/1
  I0_re_prl/1 -> Divide2/1
  I0_im_prl/1 -> Divide3/1
  K_I0_prl_re/1 -> Iph_add_3I0K1/3
  K_I0_prl_im/1 -> Iph_add_3I0K1/4
  K_I0_re/1 -> Iph_add_3I0K/3
  K_I0_im/1 -> Iph_add_3I0K/4
  Divide3/1 -> Iph_add_3I0K1/2
  Divide2/1 -> Iph_add_3I0K1/1
  Divide1/1 -> Iph_add_3I0K/2
  Divide/1 -> Iph_add_3I0K/1
  Iph_add_3I0K/1 -> Add/2
  Iph_add_3I0K/2 -> Add1/2
  Add/1 -> Add2/1
  Iph_add_3I0K1/1 -> Add2/2
  Iph_add_3I0K1/2 -> Add3/2
  Add1/1 -> Add3/1
  I_im/1 -> orto_DIV_orto/4, Add1/1
  I_re/1 -> orto_DIV_orto/3, Add/1
  U_re/1 -> orto_DIV_orto1/1, orto_DIV_orto/1
  U_im/1 -> orto_DIV_orto1/2, orto_DIV_orto/2
  Add3/1 -> orto_DIV_orto1/4
  Add2/1 -> orto_DIV_orto1/3
  orto_DIV_orto1/2 -> X_comp/1, ORTOTOMODULE/2
  orto_DIV_orto1/1 -> R_comp/1, ORTOTOMODULE/1
  orto_DIV_orto/2 -> X/1, ORTOTOMODULE1/2
  orto_DIV_orto/1 -> R/1, ORTOTOMODULE1/1
  ORTOTOMODULE/1 -> Z_comp/1
  ORTOTOMODULE1/1 -> Z/1

== system mylib/264_DZ_trans_st_v1/z_calc_ph_line19/Z_lin/Z_ab ==
  U_ph1_re : Inport
  U_ph1_im : Inport  Port=2
  U_ph2_re : Inport  Port=3
  U_ph2_im : Inport  Port=4
  I_ph1_re : Inport  Port=5
  I_ph1_im : Inport  Port=6
  I_ph2_re : Inport  Port=7
  I_ph2_im : Inport  Port=8
  det_K2 : Inport  Port=9
  Add{,1,4..5} (4 alike) : Sum  Inputs=+-
  Add2 : Sum
  Add3 : Sum
  Constant : Constant  Value=0
  Constant1 : Constant  Value=-1
  Divide : Product  Inputs=*/
  Divide1 : Product  Inputs=*/
  Divide2 : Product  Inputs=**
  Divide3 : Product  Inputs=**
  Switch : Switch  Criteria=u2 > Threshold
  Switch1 : Switch  Criteria=u2 > Threshold
  U_ph1_div_I_lin : $bdroot/orto_DIV_orto  SystemSampleTime=-1  Latency=0  AutoFrameSizeCalculation=off
  U_ph2_div_I_lin : $bdroot/orto_DIV_orto  SystemSampleTime=-1  Latency=0  AutoFrameSizeCalculation=off
  Z_lin : $bdroot/ORTOTOMODULE  SystemSampleTime=-1  Latency=0  AutoFrameSizeCalculation=off
  Z_sum : $bdroot/ORTOTOMODULE  SystemSampleTime=-1  Latency=0  AutoFrameSizeCalculation=off
  turn_90deg : $bdroot/orto_MUL_orto  SystemSampleTime=-1  Latency=0  AutoFrameSizeCalculation=off
  R : Outport
  X : Outport  Port=2
  wires:
  I_ph2_re/1 -> Add/2
  I_ph1_re/1 -> Add/1
  I_ph1_im/1 -> Add1/1
  I_ph2_im/1 -> Add1/2
  Add1/1 -> U_ph1_div_I_lin/4, U_ph2_div_I_lin/4
  Add/1 -> U_ph1_div_I_lin/3, U_ph2_div_I_lin/3
  U_ph1_re/1 -> U_ph1_div_I_lin/1
  U_ph1_im/1 -> U_ph1_div_I_lin/2
  U_ph2_re/1 -> U_ph2_div_I_lin/1
  U_ph2_im/1 -> U_ph2_div_I_lin/2
  U_ph1_div_I_lin/1 -> Add4/1, Add2/1
  U_ph2_div_I_lin/1 -> Add4/2, Add2/2
  U_ph1_div_I_lin/2 -> Add5/1, Add3/1
  U_ph2_div_I_lin/2 -> Add5/2, Add3/2
  Add4/1 -> Switch1/3, Z_lin/1
  Add5/1 -> Switch/3, Z_lin/2
  Add2/1 -> Divide1/1, Z_sum/1
  Add3/1 -> Divide/1, Z_sum/2
  Z_sum/1 -> Divide1/2, Divide/2
  Constant/1 -> turn_90deg/3
  Constant1/1 -> turn_90deg/4
  Divide/1 -> turn_90deg/2
  Divide1/1 -> turn_90deg/1
  turn_90deg/2 -> Divide2/2
  Divide2/1 -> Switch/1
  Z_lin/1 -> Divide2/1, Divide3/1
  turn_90deg/1 -> Divide3/2
  Divide3/1 -> Switch1/1
  det_K2/1 -> Switch1/2, Switch/2
  Switch/1 -> X/1
  Switch1/1 -> R/1

== system mylib/264_DZ_trans_st_v1/z_calc_ph_line19/Z_lin/Z_bc ==
  U_ph1_re : Inport
  U_ph1_im : Inport  Port=2
  U_ph2_re : Inport  Port=3
  U_ph2_im : Inport  Port=4
  I_ph1_re : Inport  Port=5
  I_ph1_im : Inport  Port=6
  I_ph2_re : Inport  Port=7
  I_ph2_im : Inport  Port=8
  det_K2 : Inport  Port=9
  Add{,1,4..5} (4 alike) : Sum  Inputs=+-
  Add2 : Sum
  Add3 : Sum
  Constant : Constant  Value=0
  Constant1 : Constant  Value=-1
  Divide : Product  Inputs=*/
  Divide1 : Product  Inputs=*/
  Divide2 : Product  Inputs=**
  Divide3 : Product  Inputs=**
  Switch : Switch  Criteria=u2 > Threshold
  Switch1 : Switch  Criteria=u2 > Threshold
  U_ph1_div_I_lin : $bdroot/orto_DIV_orto  SystemSampleTime=-1  Latency=0  AutoFrameSizeCalculation=off
  U_ph2_div_I_lin : $bdroot/orto_DIV_orto  SystemSampleTime=-1  Latency=0  AutoFrameSizeCalculation=off
  Z_lin : $bdroot/ORTOTOMODULE  SystemSampleTime=-1  Latency=0  AutoFrameSizeCalculation=off
  Z_sum : $bdroot/ORTOTOMODULE  SystemSampleTime=-1  Latency=0  AutoFrameSizeCalculation=off
  turn_90deg : $bdroot/orto_MUL_orto  SystemSampleTime=-1  Latency=0  AutoFrameSizeCalculation=off
  R : Outport
  X : Outport  Port=2
  wires:
  I_ph2_re/1 -> Add/2
  I_ph1_re/1 -> Add/1
  I_ph1_im/1 -> Add1/1
  I_ph2_im/1 -> Add1/2
  Add1/1 -> U_ph1_div_I_lin/4, U_ph2_div_I_lin/4
  Add/1 -> U_ph1_div_I_lin/3, U_ph2_div_I_lin/3
  U_ph1_re/1 -> U_ph1_div_I_lin/1
  U_ph1_im/1 -> U_ph1_div_I_lin/2
  U_ph2_re/1 -> U_ph2_div_I_lin/1
  U_ph2_im/1 -> U_ph2_div_I_lin/2
  U_ph1_div_I_lin/1 -> Add4/1, Add2/1
  U_ph2_div_I_lin/1 -> Add4/2, Add2/2
  U_ph1_div_I_lin/2 -> Add5/1, Add3/1
  U_ph2_div_I_lin/2 -> Add5/2, Add3/2
  Add4/1 -> Switch1/3, Z_lin/1
  Add5/1 -> Switch/3, Z_lin/2
  Add2/1 -> Divide1/1, Z_sum/1
  Add3/1 -> Divide/1, Z_sum/2
  Z_sum/1 -> Divide1/2, Divide/2
  Constant/1 -> turn_90deg/3
  Constant1/1 -> turn_90deg/4
  Divide/1 -> turn_90deg/2
  Divide1/1 -> turn_90deg/1
  turn_90deg/2 -> Divide2/2
  Divide2/1 -> Switch/1
  Z_lin/1 -> Divide2/1, Divide3/1
  turn_90deg/1 -> Divide3/2
  Divide3/1 -> Switch1/1
  det_K2/1 -> Switch1/2, Switch/2
  Switch/1 -> X/1
  Switch1/1 -> R/1

== system mylib/264_DZ_trans_st_v1/z_calc_ph_line19/Z_lin/Z_ca ==
  U_ph1_re : Inport
  U_ph1_im : Inport  Port=2
  U_ph2_re : Inport  Port=3
  U_ph2_im : Inport  Port=4
  I_ph1_re : Inport  Port=5
  I_ph1_im : Inport  Port=6
  I_ph2_re : Inport  Port=7
  I_ph2_im : Inport  Port=8
  det_K2 : Inport  Port=9
  Add{,1,4..5} (4 alike) : Sum  Inputs=+-
  Add2 : Sum
  Add3 : Sum
  Constant : Constant  Value=0
  Constant1 : Constant  Value=-1
  Divide : Product  Inputs=*/
  Divide1 : Product  Inputs=*/
  Divide2 : Product  Inputs=**
  Divide3 : Product  Inputs=**
  Switch : Switch  Criteria=u2 > Threshold
  Switch1 : Switch  Criteria=u2 > Threshold
  U_ph1_div_I_lin : $bdroot/orto_DIV_orto  SystemSampleTime=-1  Latency=0  AutoFrameSizeCalculation=off
  U_ph2_div_I_lin : $bdroot/orto_DIV_orto  SystemSampleTime=-1  Latency=0  AutoFrameSizeCalculation=off
  Z_lin : $bdroot/ORTOTOMODULE  SystemSampleTime=-1  Latency=0  AutoFrameSizeCalculation=off
  Z_sum : $bdroot/ORTOTOMODULE  SystemSampleTime=-1  Latency=0  AutoFrameSizeCalculation=off
  turn_90deg : $bdroot/orto_MUL_orto  SystemSampleTime=-1  Latency=0  AutoFrameSizeCalculation=off
  R : Outport
  X : Outport  Port=2
  wires:
  I_ph2_re/1 -> Add/2
  I_ph1_re/1 -> Add/1
  I_ph1_im/1 -> Add1/1
  I_ph2_im/1 -> Add1/2
  Add1/1 -> U_ph1_div_I_lin/4, U_ph2_div_I_lin/4
  Add/1 -> U_ph1_div_I_lin/3, U_ph2_div_I_lin/3
  U_ph1_re/1 -> U_ph1_div_I_lin/1
  U_ph1_im/1 -> U_ph1_div_I_lin/2
  U_ph2_re/1 -> U_ph2_div_I_lin/1
  U_ph2_im/1 -> U_ph2_div_I_lin/2
  U_ph1_div_I_lin/1 -> Add4/1, Add2/1
  U_ph2_div_I_lin/1 -> Add4/2, Add2/2
  U_ph1_div_I_lin/2 -> Add5/1, Add3/1
  U_ph2_div_I_lin/2 -> Add5/2, Add3/2
  Add4/1 -> Switch1/3, Z_lin/1
  Add5/1 -> Switch/3, Z_lin/2
  Add2/1 -> Divide1/1, Z_sum/1
  Add3/1 -> Divide/1, Z_sum/2
  Z_sum/1 -> Divide1/2, Divide/2
  Constant/1 -> turn_90deg/3
  Constant1/1 -> turn_90deg/4
  Divide/1 -> turn_90deg/2
  Divide1/1 -> turn_90deg/1
  turn_90deg/2 -> Divide2/2
  Divide2/1 -> Switch/1
  Z_lin/1 -> Divide2/1, Divide3/1
  turn_90deg/1 -> Divide3/2
  Divide3/1 -> Switch1/1
  det_K2/1 -> Switch1/2, Switch/2
  Switch/1 -> X/1
  Switch1/1 -> R/1
